simulink model "Brain_Khoo"  (Simulink 6.4)
settings: Solver=ode45  StartTime=0.0  StopTime=10.0  RelTol=1e-3
values from neighbouring files (symbols this model uses):
  h = 0.0183    [Brain_Khoo_IC.m]    (also in Gas_Exchange_IC.m; Respiratory_IC.m)
  MRbCO2 = 0.0517    [Brain_Khoo_IC.m]    (also in Gas_Exchange_IC.m; Respiratory_IC.m)
  PbCO2IC = 48.2858    [Brain_Khoo_IC.m]    (also in Gas_Exchange_IC.m; Respiratory_IC.m = 48.5383)
  QdBo = 0.8333    [Brain_Khoo_IC.m]    (also in Gas_Exchange_IC.m; Respiratory_IC.m)
  SbCO2 = 0.3600    (= 0.36)    [Brain_Khoo_IC.m]    (also in Gas_Exchange_IC.m; Respiratory_IC.m)
  SCO2 = 0.0043    [Brain_Khoo_IC.m]    (also in Gas_Exchange_IC.m; Respiratory_IC.m)
settings Model: LastModifiedBy=CLM
settings OptimizationCC: BlockReduction=off  BooleanDataType=off
settings DebuggingCC: SolverPrmCheckMsg=none  StrictBusMsg=None
settings HardwareCC: TargetUnknown=on

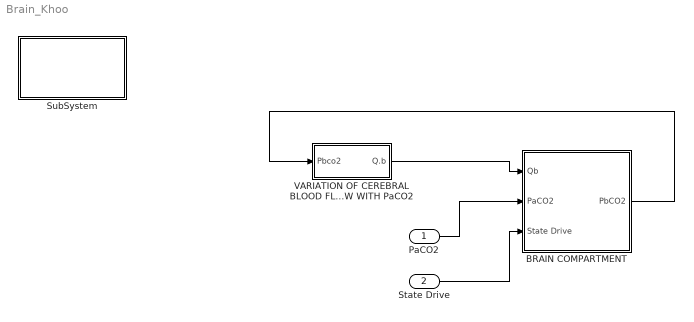
== system Brain_Khoo ==
  PaCO2 : Inport
  State Drive : Inport  Port=2
  BRAIN COMPARTMENT : Subsystem
  SubSystem : Subsystem
      settings: OpenFcn=Brain_Khoo_IC
      mask Display: disp('"double click here"\n to load \nBrain_Khoo \ninitial values');
  VARIATION OF CEREBRAL BLOOD FLOW WITH PaCO2 : Subsystem
  wires:
  VARIATION OF CEREBRAL BLOOD FLOW WITH PaCO2/1(Q.b) -> BRAIN COMPARTMENT/1(Qb)
  BRAIN COMPARTMENT/1(PbCO2) -> VARIATION OF CEREBRAL BLOOD FLOW WITH PaCO2/1(Pbco2)
  PaCO2/1 -> BRAIN COMPARTMENT/2(PaCO2)
  State Drive/1 -> BRAIN COMPARTMENT/3(State Drive)

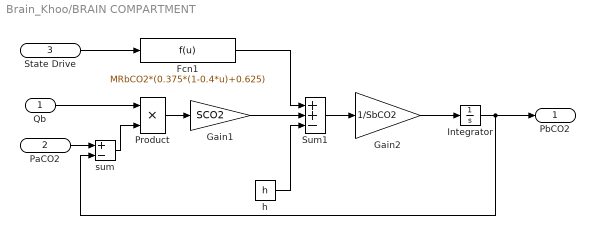
== system Brain_Khoo/BRAIN COMPARTMENT ==
  Qb : Inport
  PaCO2 : Inport  Port=2
  State Drive : Inport  Port=3
  Fcn1 : Fcn  Expr=MRbCO2*(0.375*(1-0.4*u)+0.625)
  Gain1 : Gain  Gain=SCO2  SaturateOnIntegerOverflow=on
  Gain2 : Gain  Gain=1/SbCO2  SaturateOnIntegerOverflow=on
  Integrator : Integrator  InitialCondition=PbCO2IC
  Product : Product  Inputs=**  SaturateOnIntegerOverflow=on  RndMeth=Zero  InputSameDT=on
  Sum1 : Sum  Inputs=++-  SaturateOnIntegerOverflow=on  InputSameDT=on
  h : Constant  Value=h  OutDataType=sfix(16)  ConRadixGroup=Use specified scaling  OutScaling=2^0  SampleTime=inf  FramePeriod=inf
  sum : Sum  Inputs=+-  SaturateOnIntegerOverflow=on  InputSameDT=on
  PbCO2 : Outport
  wires:
  Fcn1/1 -> Sum1/1
  Product/1 -> Gain1/1
  Gain2/1 -> Integrator/1
  Qb/1 -> Product/1
  h/1 -> Sum1/3
  sum/1 -> Product/2
  PaCO2/1 -> sum/1
  Sum1/1 -> Gain2/1
  Gain1/1 -> Sum1/2
  State Drive/1 -> Fcn1/1
  Integrator/1 -> sum/2, PbCO2/1

== system Brain_Khoo/SubSystem ==

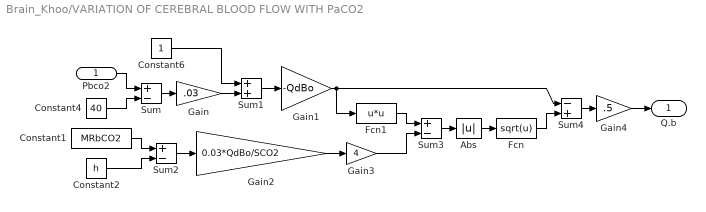
== system Brain_Khoo/VARIATION OF CEREBRAL BLOOD FLOW WITH PaCO2 ==
  Pbco2 : Inport
  Abs : Abs  SaturateOnIntegerOverflow=on  SampleTime=-1
  Constant1 : Constant  Value=MRbCO2  OutDataType=sfix(16)  ConRadixGroup=Use specified scaling  OutScaling=2^0  SampleTime=inf  FramePeriod=inf
  Constant2 : Constant  Value=h  OutDataType=sfix(16)  ConRadixGroup=Use specified scaling  OutScaling=2^0  SampleTime=inf  FramePeriod=inf
  Constant4 : Constant  Value=40  OutDataType=sfix(16)  ConRadixGroup=Use specified scaling  OutScaling=2^0  SampleTime=inf  FramePeriod=inf
  Constant6 : Constant  Value=1  OutDataType=sfix(16)  ConRadixGroup=Use specified scaling  OutScaling=2^0  SampleTime=inf  FramePeriod=inf
  Fcn : Fcn  Expr=sqrt(u)
  Fcn1 : Fcn  Expr=u*u
  Gain : Gain  Gain=.03  SaturateOnIntegerOverflow=on
  Gain1 : Gain  Gain=-QdBo  SaturateOnIntegerOverflow=on
  Gain2 : Gain  Gain=0.03*QdBo/SCO2  SaturateOnIntegerOverflow=on
  Gain3 : Gain  Gain=4  SaturateOnIntegerOverflow=on
  Gain4 : Gain  Gain=.5  SaturateOnIntegerOverflow=on
  Sum : Sum  Inputs=+-  SaturateOnIntegerOverflow=on  InputSameDT=on
  Sum1 : Sum  SaturateOnIntegerOverflow=on  InputSameDT=on
  Sum2 : Sum  Inputs=+-  SaturateOnIntegerOverflow=on  InputSameDT=on
  Sum3 : Sum  Inputs=+-  SaturateOnIntegerOverflow=on  InputSameDT=on
  Sum4 : Sum  Inputs=-+  SaturateOnIntegerOverflow=on  InputSameDT=on
  Q.b : Outport
  wires:
  Gain4/1 -> Q.b/1
  Abs/1 -> Fcn/1
  Sum3/1 -> Abs/1
  Gain1/1 -> Fcn1/1, Sum4/1
  Fcn1/1 -> Sum3/1
  Pbco2/1 -> Sum/1
  Constant4/1 -> Sum/2
  Sum/1 -> Gain/1
  Gain/1 -> Sum1/2
  Constant6/1 -> Sum1/1
  Sum1/1 -> Gain1/1
  Constant1/1 -> Sum2/1
  Constant2/1 -> Sum2/2
  Sum2/1 -> Gain2/1
  Gain2/1 -> Gain3/1
  Gain3/1 -> Sum3/2
  Fcn/1 -> Sum4/2
  Sum4/1 -> Gain4/1
